simulink subsystem "wheelSpeed"  (R2023b)
settings: Solver=VariableStepAuto  StartTime=0.0  StopTime=10.0  RelTol=1e-3
libraries: Raptor_lib x5, wheelSpeed_lib x4
settings Model: Creator=serga  LastModifiedBy=serga
settings OptimizationCC: ReuseModelBlockBuffer=off

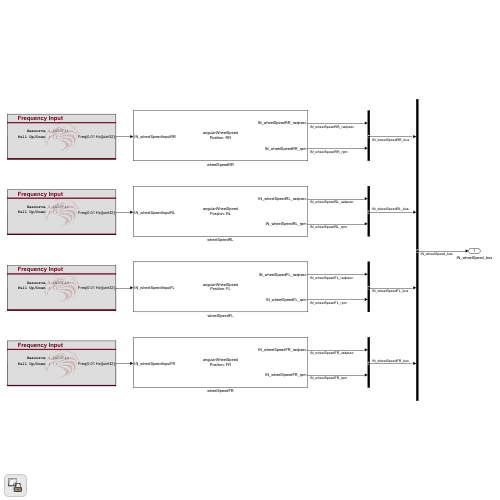
[thumbnail: Simulink's stored preview of the top-level diagram]
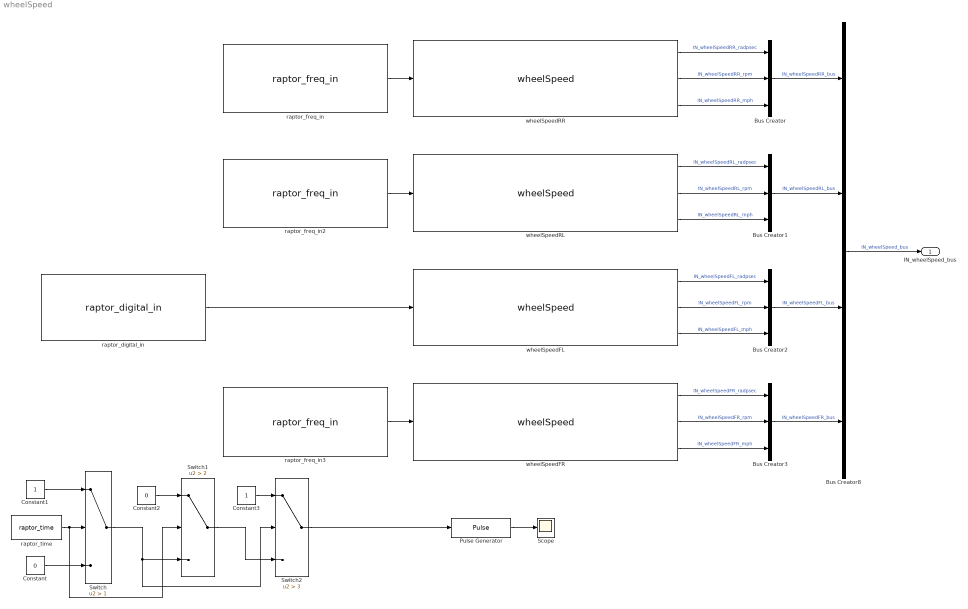
== system wheelSpeed ==
  Bus Creator{,1..3} (4 alike) : BusCreator  Inputs=3
  Bus Creator8 : BusCreator  Inputs=4
  Constant : Constant  Value=0
  Constant1 : Constant
  Constant2 : Constant  Value=0
  Constant3 : Constant
  Pulse Generator : DiscretePulseGenerator  PulseType=Time based  TimeSource=Use external signal  Period=10  PulseWidth=5
  Scope : Scope
  Switch : Switch  Criteria=u2 > Threshold  Threshold=1  SaturateOnIntegerOverflow=off  InputSameDT=off
  Switch1 : Switch  Criteria=u2 > Threshold  Threshold=2  SaturateOnIntegerOverflow=off  InputSameDT=off
  Switch2 : Switch  Criteria=u2 > Threshold  Threshold=3  SaturateOnIntegerOverflow=off  InputSameDT=off
  raptor_digital_in : Raptor_lib/Input & Output/raptor_digital_in  resourceValues=WAKE_INPUT1|INPUT33|INPUT34|INPUT35|INPUT36|INPUT37|INPUT38|INPUT39|INPUT40|(None)  resource=INPUT36  pullUDValues=2.6k PU  pullUD=2.6k PU  upperThres='RAPTOR MASK DEFAULT'  lowerThres='RAPTOR MASK DEFAULT'
      settings: SourceProductName=Raptor
  raptor_freq_in : Raptor_lib/Input & Output/raptor_freq_in  minFreq=1  resourceValues=INPUT41|INPUT42|INPUT43|INPUT44|INPUT45|(None)  resource=INPUT42  pullUDValues=[]  pullUD=[]  interfaceValues=[]  interface=[]  hasDuty=off  hasEdgeCount=off
      settings: SourceProductName=Raptor
  raptor_freq_in2 : Raptor_lib/Input & Output/raptor_freq_in  minFreq=1  resourceValues=INPUT41|INPUT42|INPUT43|INPUT44|INPUT45|(None)  resource=INPUT45  pullUDValues=[]  pullUD=[]  interfaceValues=[]  interface=[]  hasDuty=off  hasEdgeCount=off
      settings: SourceProductName=Raptor
  raptor_freq_in3 : Raptor_lib/Input & Output/raptor_freq_in  minFreq=1  resourceValues=INPUT41|INPUT42|INPUT43|INPUT44|INPUT45|(None)  resource=INPUT44  pullUDValues=[]  pullUD=[]  interfaceValues=[]  interface=[]  hasDuty=off  hasEdgeCount=off
      settings: SourceProductName=Raptor
  raptor_time : Raptor_lib/Triggers/raptor_time  unit=milliseconds
      settings: SourceProductName=Raptor
  wheelSpeedFL : wheelSpeed_lib/wheelSpeed  pos='FL'
  wheelSpeedFR : wheelSpeed_lib/wheelSpeed  pos='FR'
  wheelSpeedRL : wheelSpeed_lib/wheelSpeed  pos='RL'
  wheelSpeedRR : wheelSpeed_lib/wheelSpeed  pos='RR'
  IN_wheelSpeed_bus : Outport
  wires:
  Bus Creator2/1 -> Bus Creator8/3  "IN_wheelSpeedFL_bus"
  Bus Creator1/1 -> Bus Creator8/2  "IN_wheelSpeedRL_bus"
  Bus Creator8/1 -> IN_wheelSpeed_bus/1  "IN_wheelSpeed_bus"
  Bus Creator3/1 -> Bus Creator8/4  "IN_wheelSpeedFR_bus"
  Bus Creator/1 -> Bus Creator8/1  "IN_wheelSpeedRR_bus"
  raptor_freq_in/1 -> wheelSpeedRR/1
  raptor_freq_in2/1 -> wheelSpeedRL/1
  raptor_digital_in/1 -> wheelSpeedFL/1
  raptor_freq_in3/1 -> wheelSpeedFR/1
  wheelSpeedRR/1 -> Bus Creator/1  "IN_wheelSpeedRR_radpsec"
  wheelSpeedRR/2 -> Bus Creator/2  "IN_wheelSpeedRR_rpm"
  wheelSpeedRL/1 -> Bus Creator1/1  "IN_wheelSpeedRL_radpsec"
  wheelSpeedRL/2 -> Bus Creator1/2  "IN_wheelSpeedRL_rpm"
  wheelSpeedFL/1 -> Bus Creator2/1  "IN_wheelSpeedFL_radpsec"
  wheelSpeedFL/2 -> Bus Creator2/2  "IN_wheelSpeedFL_rpm"
  wheelSpeedFR/1 -> Bus Creator3/1  "IN_wheelSpeedFR_radpsec"
  wheelSpeedFR/2 -> Bus Creator3/2  "IN_wheelSpeedFR_rpm"
  wheelSpeedRR/3 -> Bus Creator/3  "IN_wheelSpeedRR_mph"
  wheelSpeedRL/3 -> Bus Creator1/3  "IN_wheelSpeedRL_mph"
  wheelSpeedFL/3 -> Bus Creator2/3  "IN_wheelSpeedFL_mph"
  wheelSpeedFR/3 -> Bus Creator3/3  "IN_wheelSpeedFR_mph"
  Pulse Generator/1 -> Scope/1
  raptor_time/1 -> Switch/2, Switch1/2
  Constant/1 -> Switch/3
  Constant1/1 -> Switch/1
  Switch/1 -> Switch1/3, Switch2/2
  Constant2/1 -> Switch1/1
  Switch1/1 -> Switch2/3
  Constant3/1 -> Switch2/1
  Switch2/1 -> Pulse Generator/1
